simulink model "LTI_System"  (R2024b)
settings: Solver=VariableStepAuto  StartTime=0.0  StopTime=2000.0  RelTol=1e-3
values from neighbouring files (symbols this model uses):
  A = A0    [buildGainGrid.m]    (also in rovHoverModel.m = [ zeros(6),       eye(6))
  B = B0    [buildGainGrid.m]    (also in makeFeedForwardTau.m = p.rho * p.g * p.volume; rovHoverModel.m = [ zeros(6))
  C_integration = C(1:6,:)    [main_hover_controller.m]
  C_real = C_real(meas_idx, :)    [main_hover_controller.m]
  D = diag(p.D_lin) + diag(p.D_quad .* abs(nu))    [computeDynamicsSimple.m]    (also in makeFeedForwardTau.m = D_lin + D_quad; rovHoverModel.m = zeros(12,6))
  Ki = Kfull(:, n+1:end)    [designHoverController.m]    (also in designHoverControllerAtTrim.m)
  Kx = Kfull(:, 1:n)    [designHoverController.m]    (also in designHoverControllerAtTrim.m)
  L = 0.5    [animateTrajectoryGIF.m]    (also in buildMixingMatrix.m = 0.575; main_hover_controller.m = lqe(A, G, C_real, Qn, Rn); test_linear_hover.m = 400; visualizeTrajectory.m = 1)
settings Model: Creator=eirikvarnes  LastModifiedBy=eirikvarnes
settings DataIOCC: ReturnWorkspaceOutputs=off

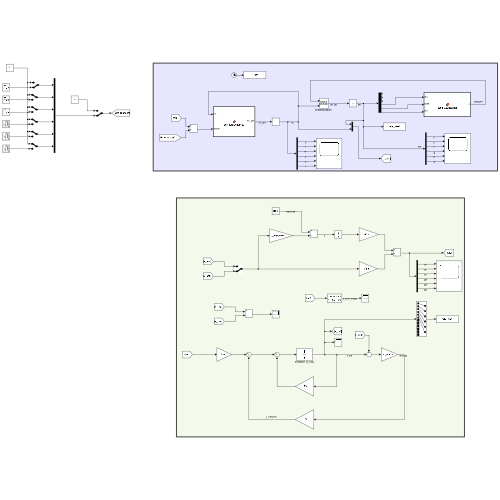
[thumbnail: Simulink's stored preview of the top-level diagram]
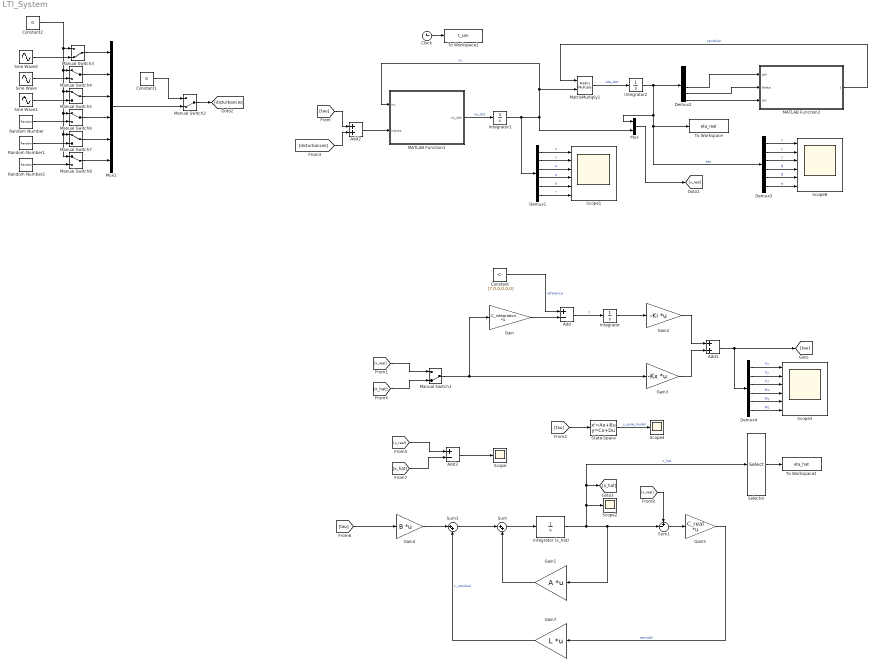
== system LTI_System ==
  Add : Sum  Inputs=+-
  Add1 : Sum
  Add2 : Sum
  Add3 : Sum  Inputs=+-
  Clock : Clock
  Constant : Constant  Value=[7,0,0,0,0,0]
  Constant1 : Constant  Value=0
  Constant2 : Constant  Value=0
  Demux{1..4} (4 alike) : Demux  Outputs=6
  Gain : Gain  Gain=C_integration  Multiplication=Matrix(K*u)
  Gain1 : Gain  Gain=A  Multiplication=Matrix(K*u)
  Gain2 : Gain  Gain=-Ki  Multiplication=Matrix(K*u)
  Gain3 : Gain  Gain=-Kx  Multiplication=Matrix(K*u)
  Gain4 : Gain  Gain=B  Multiplication=Matrix(K*u)
  Gain5 : Gain  Gain=C_real  Multiplication=Matrix(K*u)
  Gain7 : Gain  Gain=L  Multiplication=Matrix(K*u)
  Integrator : Integrator
  Integrator (x_hat) : Integrator
  Integrator1 : Integrator
  Integrator2 : Integrator
  MATLAB Function1 : MATLAB Function  TreatAsAtomicUnit=on
  MATLAB Function2 : MATLAB Function  TreatAsAtomicUnit=on
  Manual Switch1 : ManualSwitch  CurrentSetting=0
  Manual Switch2 : ManualSwitch  CurrentSetting=0
  Manual Switch3 : ManualSwitch  CurrentSetting=0
  Manual Switch{4..8} (5 alike) : ManualSwitch
  MatrixMultiply1 : Product  Multiplication=Matrix(*)
  Mux : Mux  Inputs=2
  Mux1 : Mux  Inputs=6
  Random Number : RandomNumber  Variance=0.01  SampleTime=0.1
  Random Number1 : RandomNumber  Variance=0.01  SampleTime=0.1
  Random Number2 : RandomNumber  Variance=0.01  SampleTime=0.1
  Scope : Scope
  Scope1 : Scope  NumInputPorts=6
  Scope2 : Scope
  Scope3 : Scope  NumInputPorts=6
  Scope4 : Scope
  Scope8 : Scope  NumInputPorts=6
  Selector : Selector  InputPortWidth=12  IndexOptions=Index vector (dialog)  Indices=[1 2 3 4 5 6]  OutputSizes=1
  Sine Wave : Sin  Amplitude=0.1  Frequency=0.05  SampleTime=0
  Sine Wave1 : Sin  Amplitude=0.1  Frequency=0.08  SampleTime=0
  Sine Wave2 : Sin  Amplitude=0.1  Frequency=0.05  SampleTime=0
  State-Space : StateSpace  A=A  B=B  C=eye(12)  D=D  InitialCondition=0
  Sum : Sum  Inputs=|++
  Sum1 : Sum  Inputs=+-|
  Sum3 : Sum  Inputs=|++
  To Workspace : ToWorkspace  VariableName=eta_real  SampleTime=-1
  To Workspace1 : ToWorkspace  VariableName=t_sim  SampleTime=-1
  To Workspace2 : ToWorkspace  VariableName=eta_hat  SampleTime=-1
  wires:
  Integrator1/1 -> Mux/2, MATLAB Function1/1(nu), MatrixMultiply1/2, Demux1/1  "nu"
  Demux2/6 -> MATLAB Function2/3(psi)
  MATLAB Function1/1(nu_dot) -> Integrator1/1  "nu_dot"
  Demux2/4 -> MATLAB Function2/1(phi)
  Integrator2/1 -> To Workspace/1, Demux3/1, Mux/1, Demux2/1  "eta"
  Demux2/5 -> MATLAB Function2/2(theta)
  MatrixMultiply1/1 -> Integrator2/1  "eta_dot"
  MATLAB Function2/1(J) -> MatrixMultiply1/1  "Jacobian"
  Constant/1 -> Add/1  "reference"
  Gain/1 -> Add/2
  Manual Switch1/1 -> Gain/1, Gain3/1
  Add/1 -> Integrator/1  "z"
  Integrator/1 -> Gain2/1
  Gain3/1 -> Add1/2
  Gain2/1 -> Add1/1
  Integrator (x_hat)/1 -> Selector/1, [x_hat], Scope2/1, Sum1/2, Gain1/1  "x_hat"
  Sum/1 -> Integrator (x_hat)/1
  Gain1/1 -> Sum/2
  Gain4/1 -> Sum3/1
  Gain7/1 -> Sum3/2  "L_residual"
  Sum3/1 -> Sum/1
  Add1/1 -> [tau], Demux4/1
  [tau] -> Gain4/1
  [tau] -> State-Space/1
  Mux/1 -> [x_real]
  [x_real] -> Manual Switch1/1
  [tau] -> Add2/1
  [disturbances] -> Add2/2
  Add2/1 -> MATLAB Function1/2(inputs)
  Manual Switch2/1 -> [disturbances]
  Mux1/1 -> Manual Switch2/2
  Constant1/1 -> Manual Switch2/1
  Constant2/1 -> Manual Switch8/1, Manual Switch7/1, Manual Switch6/1, Manual Switch5/1, Manual Switch4/1, Manual Switch3/1
  Manual Switch4/1 -> Mux1/2
  Manual Switch3/1 -> Mux1/1
  Manual Switch5/1 -> Mux1/3
  Manual Switch6/1 -> Mux1/4
  Manual Switch7/1 -> Mux1/5
  Manual Switch8/1 -> Mux1/6
  Sine Wave2/1 -> Manual Switch3/2
  Sine Wave/1 -> Manual Switch4/2
  Sine Wave1/1 -> Manual Switch5/2
  Random Number/1 -> Manual Switch6/2
  Random Number1/1 -> Manual Switch7/2
  Random Number2/1 -> Manual Switch8/2
  [x_hat] -> Manual Switch1/2
  [x_real] -> Add3/1
  [x_hat] -> Add3/2
  Add3/1 -> Scope/1
  Demux4/1 -> Scope3/1  "Fx"
  Demux4/6 -> Scope3/6  "Mz"
  Demux4/4 -> Scope3/4  "Mx"
  Demux4/3 -> Scope3/3  "Fz"
  Demux4/2 -> Scope3/2  "Fy"
  Demux4/5 -> Scope3/5  "My"
  [x_real] -> Sum1/1
  Gain5/1 -> Gain7/1  "resiudal"
  Sum1/1 -> Gain5/1
  Clock/1 -> To Workspace1/1
  Demux1/1 -> Scope1/1  "u"
  Demux1/6 -> Scope1/6  "r"
  Demux1/4 -> Scope1/4  "p"
  Demux1/3 -> Scope1/3  "w"
  Demux1/2 -> Scope1/2  "v"
  Demux1/5 -> Scope1/5  "q"
  Demux3/5 -> Scope8/5  "θ"
  Demux3/4 -> Scope8/4  "ϕ"
  Demux3/2 -> Scope8/2  "y"
  Demux3/6 -> Scope8/6  "ψ"
  Demux3/3 -> Scope8/3  "z"
  Demux3/1 -> Scope8/1  "x"
  Selector/1 -> To Workspace2/1
  State-Space/1 -> Scope4/1  "y_pure_model"

== matlab function LTI_System/MATLAB Function1 ==
  data: nu input size=[6 1]; inputs input; nu_dot output size=[6 1]
function nu_dot = computeDynamics(nu, inputs)
% computeDynamics  1st‐order dynamics with added‐mass & damping only
%   nu_dot = M_R^{-1} * (tau_ff - D*nu)
%
%   Inputs nu and tau_ff must both be 6-by-1 vectors.

  %#codegen
  % Verify inputs are 6-by-1
  assert(all(size(nu)==[6,1]),  'computeDynamics:InvalidInput', 'nu must be 6-by-1');
  assert(all(size(inputs)==[6,1]), 'computeDynamics:InvalidInput', 'tau_ff must be 6-by-1');

  % Pull in parameters
  params = rovParameters();

  % Total mass + added‐mass
  M_rb = [params.mass*eye(3), zeros(3);
          zeros(3),           params.I];
  M_A  = -diag([params.Ma_lin; params.Ma_rot]);
  M_R  = M_rb + M_A;

  % Damping
  D_lin  = diag(params.D_lin);
  D_quad = diag(params.D_quad .* abs(nu));
  D      = D_lin + D_quad;

  % Dynamics
  nu_dot = M_R \ (inputs - D*nu);
end

== matlab function LTI_System/MATLAB Function2 ==
  data: phi input; J output; theta input; psi input
function J = computeJacobian(phi, theta, psi)
% computeJacobian  ZYX‐Euler Jacobian with singularity clamp
%   Inputs:
%     phi, theta, psi  – Euler angles (roll, pitch, yaw), in radians
%   Output:
%     J  – 6×6 Jacobian mapping [u;v;w;p;q;r] to [xdot;ydot;zdot;phidot;thetadot;psidot]

  %#codegen
  % 1) Rotation matrix R = Rz(psi)*Ry(theta)*Rx(phi)
  cphi = cos(phi);   sphi = sin(phi);
  ctheta = cos(theta); stheta = sin(theta);
  cpsi = cos(psi);   spsi = sin(psi);

  Rz = [ cpsi, -spsi, 0;
         spsi,  cpsi, 0;
           0 ,    0 , 1 ];
  Ry = [ ctheta, 0, stheta;
            0  , 1,   0  ;
        -stheta,0, ctheta ];
  Rx = [ 1,   0  ,   0   ;
         0, cphi, -sphi ;
         0, sphi,  cphi ];
  R = Rz * Ry * Rx;

  % 2) Clamp cos(theta) away from zero to avoid singularity
  epsilon = 5e-3;                          % adjust if needed
  safe_ct = max(abs(ctheta), epsilon) * sign(ctheta);

  % 3) Build T matrix for Euler rates
  %    [phidot; thetadot; psidot] = T * [p; q; r]
  T = [ 1,      sphi*(stheta/safe_ct),   cphi*(stheta/safe_ct);
        0,            cphi,                -sphi;
        0,     sphi/safe_ct,             cphi/safe_ct ];

  % 4) Assemble full Jacobian
  J = [ R,          zeros(3,3);
        zeros(3,3), T       ];
end
